simulink model "examp1"  (Simulink 4.00)
settings: Solver=ode45  StartTime=0.0  StopTime=10.0  RelTol=1e-3
settings Model: LastModifiedBy=User

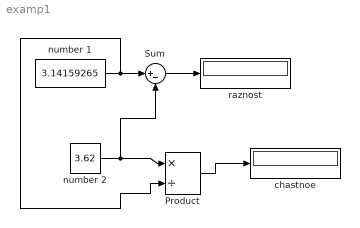
== system examp1 ==
  Product : Product  Inputs=*/  Multiplication=Element-wise(.*)  SaturateOnIntegerOverflow=on
  Sum : Sum  Inputs=|+-  SaturateOnIntegerOverflow=on
  chastnoe : Display
      settings: Format=short
  number 1 : Constant  Value=3.14159265
  number 2 : Constant  Value=3.62
  raznost : Display
      settings: Format=short
  wires:
  number 1/1 -> Sum/1, Product/2
  Sum/1 -> raznost/1
  number 2/1 -> Sum/2, Product/1
  Product/1 -> chastnoe/1
